simulink model "ZyboPWMGenTest"  (R2020a)
settings: Solver=FixedStepAuto  StartTime=0.0  StopTime=inf  FixedStep=0.001  RelTol=1e-3  EnableMultiTasking=on
libraries: zybo_lib x4, zynqlib x3, simulink x1
settings Model: Creator=Jeedella  LastModifiedBy=Jeedella
settings SolverCC: PositivePriorityOrder=on
settings OptimizationCC: EnhancedBackFolding=on  PassReuseOutputArgsAs=Individual arguments  ZeroExternalMemoryAtStartup=off  ZeroInternalMemoryAtStartup=off  MaxStackSize=64  OptimizeBlockOrder=speed  DifferentSizesBufferReuse=on  OptimizationCustomize=off  EfficientTunableParamExpr=on
settings DebuggingCC: ParameterTunabilityLossMsg=error
settings HardwareCC: ProdBitPerPointer=32  ProdBitPerSizeT=32  ProdBitPerPtrDiffT=32  ProdLargestAtomicInteger=Long  ProdLargestAtomicFloat=Double  ProdWordSize=32  ProdLongLongMode=on  ProdHWDeviceType=ARM Compatible->ARM Cortex
settings SFSimCC: MATLABDynamicMemAlloc=off
settings RTWCC: SystemTargetFile=ert.tlc  HardwareBoard=Xilinx Zynq-7000 based board  TemplateMakefile=ert_default_tmf  Toolchain=Linaro AArch32 Linux v6.3.1
settings CodeAppCC: ForceParamTrailComments=on  IgnoreCustomStorageClasses=off  OperatorAnnotations=on  SimulinkDataObjDesc=on  SFDataObjDesc=on  InsertBlockDesc=on

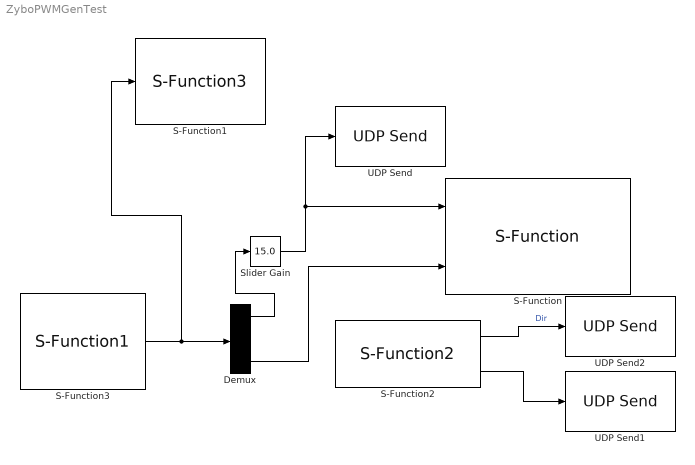
== system ZyboPWMGenTest ==
  Demux : Demux
  S-Function : zybo_lib/S-Function  PWM=0X43C30000  PERIOD=100000  MIN=0  DIR=0
      settings: SourceProductName=Zybo Library
  S-Function1 : zybo_lib/S-Function3  LEDS=0X41220008
      settings: SourceProductName=Zybo Library
  S-Function2 : zybo_lib/S-Function2  QDEC=0X43C20000
      settings: SourceProductName=Zybo Library
  S-Function3 : zybo_lib/S-Function1  SWS=0X41220000
      settings: SourceProductName=Zybo Library
  Slider Gain : simulink/Math Operations/Slider Gain  gain=15.0  low=0  high=100
  UDP Send : zynqlib/UDP Send  remoteURL='192.168.4.1'  remotePort=25004  localURL='255.255.255.255'  localPortSource=Automatically determine  localPort=-1  sendBufferSize=8192  sampletime=-1  blockPlatform=ZYNQ  separateLengthPort=0
      settings: SourceProductBaseCode=ECZYNQ7000
  UDP Send1 : zynqlib/UDP Send  remoteURL='192.168.4.1'  remotePort=25002  localURL='255.255.255.255'  localPortSource=Automatically determine  localPort=-1  sendBufferSize=8192  sampletime=-1  blockPlatform=ZYNQ  separateLengthPort=0
      settings: SourceProductBaseCode=ECZYNQ7000
  UDP Send2 : zynqlib/UDP Send  remoteURL='192.168.4.1'  remotePort=25000  localURL='255.255.255.255'  localPortSource=Automatically determine  localPort=-1  sendBufferSize=8192  sampletime=-1  blockPlatform=ZYNQ  separateLengthPort=0
      settings: SourceProductBaseCode=ECZYNQ7000
  wires:
  Demux/1 -> Slider Gain/1
  S-Function3/1 -> S-Function1/1, Demux/1
  Slider Gain/1 -> S-Function/1, UDP Send/1
  S-Function2/1 -> UDP Send2/1  "Dir"
  S-Function2/2 -> UDP Send1/1
  Demux/4 -> S-Function/2
